simulink model "simulator"  (R2025b)
settings: Solver=FixedStepAuto  StartTime=0.0  StopTime=3  FixedStep=0.01  RelTol=1e-3
values from neighbouring files (symbols this model uses):
  dt = system_params.dt    [discretize_system.m]    (also in model_init.m)
  q0 = [0; 0; 0]    [model_init.m]    (also in test_model.m = x_test(1:3))
  qdot0 = [0;0;0]    [model_init.m]
  u0 = system_params.u0(i)    [Q_tension_calc.m]    (also in Tau_tension_calc.m; model_init.m = u0_calc(q0, system_params); u0_calc.m = zeros(size(fields)))
undefined symbols (not defined in the file or in its folder): Cd, Dd, EKF_settings, P0, system_params, u0_mpc, u_dp, x0_EKF
libraries: slpidlib x5, mpclib x2
(part 2 of 2)

== matlab function simulator/Simulator/MATLAB Function2 ==
  data: x input; u input; udot input; y output; system_params input
function y = fcn(x, u, udot, system_params)

y = system_model_continous(x, u, udot, system_params);

== matlab function simulator/Simulator/Runge Kutta ==
  data: x_prev input; y output; u_k input; udot input; Ts input; system_params input
function y = fcn(x_prev, u_k, udot, Ts, system_params)
y = runge_kutta4(x_prev, u_k, udot, Ts, system_params);

== matlab function simulator/Simulator/Q_Tension ==
  data: ui input; y output; uidot input; lidot input; system_params input
function y = fcn(ui, uidot, lidot, system_params)
R_h = Rot_mat(q);
R_hxy = Rot_xy(q);
Q = zeros(3,1);
fields = fieldnames(system_params.cables);

for i = 1:numel(fields)
    cable = system_params.cables.(fields{i});
    %if i < 4
        ri = - R_h*cable.L + cable.M;
        %ri = R_h*cable.L - cable.M;
        rpli = R_h * cable.L;
        % Calc drdq
        drdq_ = drdq(q, rpli);
        
    % else
    %     ri = - R_hxy*cable.L + cable.M;
    %     ri = R_hxy*cable.L - cable.M;
    %     rpli = R_hxy * cable.L;
    %     % Calc drdq
    %     drdq_ = drdq(q, rpli);
    % 
    % end
    li = norm(ri);
    di = ri/li;
    dldq = zeros(3,1);
    for j = 1:3
        dldq(j) = di'*drdq_(:,j);
    end
    drdq_;
    lidot = dldq'*qdot;
    %lidot_check = dot(di, cross(omega, p_i));
    % numerical derivative
    eps = 1e-6;
    q_eps = q + qdot * eps;
    
    % recompute length at slightly forward time
    R_eps = Rot_mat(q_eps);
    r_eps = R_eps * cable.L -cable.M;
    l_eps = norm(r_eps);
    
    lidot_num = (l_eps - li)/eps;

    dldq_num = zeros(3,1);
    
    for j = 1:3
        dq = zeros(3,1);
        dq(j) = eps;
    
        q_eps = q + dq;
    
        % recompute rotation
        R_eps = Rot_mat(q_eps);
    
        % recompute cable vector (IMPORTANT: same definition as ri)
        %if i < 4
             ri_eps = R_eps * cable.L - cable.M;
        % else
        %     Rxy_eps = Rot_xy(q_eps);
        %     ri_eps = Rxy_eps * cable.L - cable.M;
        % end
    
        li_eps = norm(ri_eps);
    
        dldq_num(j) = (li_eps - li) / eps;
    end
    
    % Compare
    lidot;
    lidot_num;
    %disp('Analytical vs Numerical dldq:')
    %disp([dldq, dldq_num])
    
    dldq;
    di;
    drdq_;
    T = Tension(u(i), li, udot(i), lidot, system_params);
    
y = Tension(ui, li, uidot, lidot, system_params);

== matlab function simulator/Simulator/QiCalc ==
  settings: updateMethod=DISCRETE  sampleTime=dt
  data: u input; udot input; y output; q input; qdot input; system_params input
function y = fcn(u, udot, q, qdot, system_params)
y = Q_tension_calc(u, udot, q, qdot, system_params);

== matlab function simulator/Simulator/MATLAB Function ==
  data: q input; qdot input; W input; dLdq_ output; m input; g input; Lh input
function dLdq_ = dLdq_call(q, qdot, W, m, g, Lh)
    temp_struct.W = W;
    temp_struct.m = m;
    temp_struct.g = g;
    temp_struct.L_h = Lh;
    dLdq_ = dLdq(q, qdot, temp_struct);
end

== matlab function simulator/Controller/R calc ==
  data: q input; R output
function R = fcn(q)
R = Rot_mat(q);

== matlab function simulator/Controller/Q_abduction ==
  data: f input; Q output; q input; rpli input; rpmi input; R input
function Q = fcn(f, q, rpli, rpmi, R)

Q = Qi(f, q, rpli, rpmi, R);

== matlab function simulator/Controller/Q_external_rotation_upper ==
  data: f input; Q output; q input; rpli input; rpmi input; R input
function Q = fcn(f, q, rpli, rpmi, R)

Q = Qi(f, q, rpli, rpmi, R);

== matlab function simulator/Controller/Q_interal_rotation_upper ==
  data: f input; Q output; q input; rpli input; rpmi input; R input
function Q = fcn(f, q, rpli, rpmi, R)

Q = Qi(f, q, rpli, rpmi, R);

== matlab function simulator/Controller/Q_Extension ==
  data: f input; Q output; q input; rpli input; rpmi input; R input
function Q = fcn(f, q, rpli, rpmi, R)

Q = Qi(f, q, rpli, rpmi, R);

== matlab function simulator/Controller/Q_Flexion ==
  data: f input; Q output; q input; rpli input; rpmi input; R input
function Q = fcn(f, q, rpli, rpmi, R)

Q = Qi(f, q, rpli, rpmi, R);
